simulink library "CarMaker4SL"  (Simulink 8.8)
settings: Solver=ode45  StartTime=0.0  StopTime=10.0  RelTol=1e-3
libraries: simulink x1
(part 1 of 2)
settings Model: Creator=fh  LastModifiedBy=Jeder  ExtModeAutoUpdateStatusClock=off

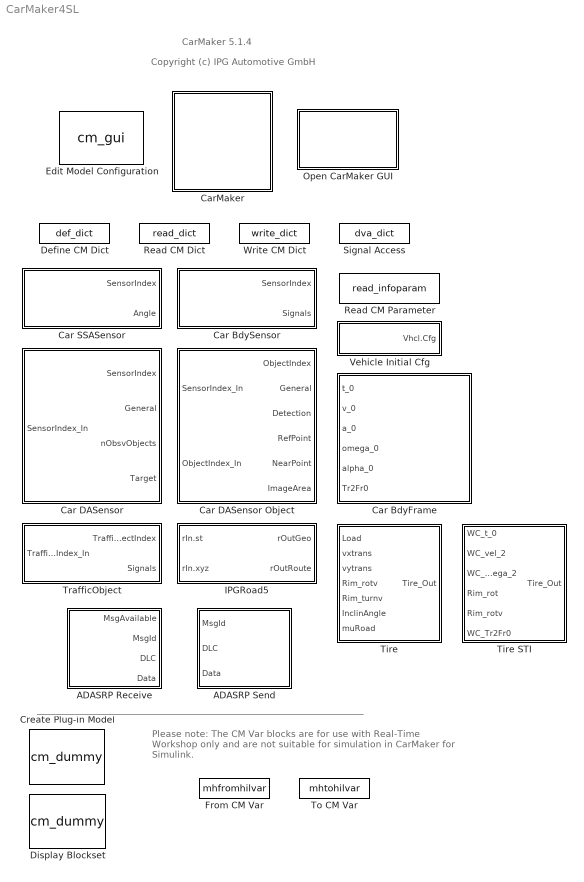
== system CarMaker4SL ==
  note: CarMaker 5.1.4
  note: Copyright (c) IPG Automotive GmbH
  note: ______________________________________________________________________
  note: Please note:
      | The CM Var blocks are for use with Real-Time Workshop only
      | and are not suitable for simulation in CarMaker for Simulink.
  ADASRP Receive : Subsystem  mask(ADASRP Receive){}
      mask help: Receive ADASP CAN message.
  ADASRP Send : Subsystem  mask(ADASRP Send){}
      mask help: Send ADASP CAN message.
  Car BdyFrame : Subsystem  mask(Body Frame){xname=[]}
      mask prompts: xname "BdyFrame name"
      mask help: Create a body frame on which sensors can be mounted.
      mask Display:
      | fprintf('<< %s >>', xname)
      | port_label('input', 1, 't_0')
      | port_label('input', 2, 'v_0')
      | port_label('input', 3, 'a_0')
      | port_label('input', 4, 'omega_0')
      | port_label('input', 5, 'alpha_0')
      | port_label('input', 6, 'Tr2Fr0')
  Car BdySensor : Subsystem  mask(CarMaker Bdy Sensor){xname=[]}
      mask prompts: xname "BdySensor name (or index)"
      mask help:
      | Read BdySensor.
      | The 'SensorIndex' outport shows either the sensor's internal index, or -1 if no BdySensor with the specified name exists.
      mask Display:
      | fprintf('<< %s >>', xname)
      | port_label('output', 1, 'SensorIndex')
      | port_label('output', 2, 'Signals')
  Car DASensor : Subsystem  mask(CarMaker Driving Assistance Sensor){xname=INPORT}
      mask prompts: xname "DASensor (name, index, or INPORT)"
      mask help:
      | Read Driving Assistance Sensor.
      | The sensor to be read may be specified in one of the following ways: 1. By giving the sensor's name. 2. By giving the sensor's numerical index. 3. By using the special name INPORT, so that the sensor's index is read from the 'si' inport.
      | The 'SensorIndex' outport shows either the sensor's index or -1 if no DASensor with the given name or index exists.
      mask Display:
      | fprintf('<< %s >>', xname)
      | port_label('input', 1, 'si')
      | port_label('output', 1, 'SensorIndex')
      | port_label('output', 2, 'General')
      | port_label('output', 3, 'nObsvObjects')
      | port_label('output', 4, 'Target')
  Car DASensor Object : Subsystem  mask(CarMaker Driving Assistance Sensor Object){xname=INPORT, ximode=Observed Objects}
      mask prompts: xname "DASensor Name (name, index, or INPORT)"; ximode "Addressed Objects"
      mask help:
      | Access sensor specific information about a traffic object.
      | The associated DASensor may be specified in one of the following ways: 1. By giving the sensor's name. 2. By giving the sensor's numerical index. 3. By using the special name INPORT, so that the sensor's index is read from the 'si' inport.
      | The object index is always read from the 'oi' inport. The 'ObjectIndex' outport shows either the object's index (world object index, see below) or -1 if no DASensor with the given name or index or no object at the given index exists.
      | You may use the special object index 99999 to select the sensor's relevant target object.
      | The object index addresses either one of the 'World Objects', i.e. all existing traffic objects, or one of the 'Observed Objects', i.e. the subset of objects inside the sensor's observation radius.
      mask TypeOptions ximode: Observed Objects | World Objects
      mask Display:
      | fprintf('<< %s >>', xname)
      | port_label('input', 1, 'si')
      | port_label('input', 2, 'oi')
      | port_label('output', 1, 'ObjectIndex')
      | port_label('output', 2, 'General')
      | port_label('output', 3, 'Detection')
      | port_label('output', 4, 'RefPoint')
      | port_label('output', 5, 'NearPoint')
      | port_label('output', 6, 'ImageArea')
  Car SSASensor : Subsystem  mask(CarMaker SideSlipAngle Sensor){xname=[]}
      mask prompts: xname "SSASensor name (or index)"
      mask help:
      | Read SideSlipAngle Sensor.
      | The 'SensorIndex' outport shows either the sensor's internal index, or -1 if no SSASensor with the specified name exists.
      mask Display:
      | fprintf('<< %s >>', xname)
      | port_label('output', 1, 'SensorIndex')
      | port_label('output', 2, 'Angle')
  CarMaker : Subsystem  TreatAsAtomicUnit=on
      mask Display: image(imread('CarMaker4SLss.bmp'));
  Create Plug-in Model : S-Function  FunctionName=cm_dummy  SFunctionDeploymentMode=off  EnableBusSupport=off  mask(Create CarMaker Plug-in Model){}
      settings: OpenFcn=cmPluginModel;
      mask Display: disp('Create\nCarMaker\nPlug-in Model');
  Define CM Dict : S-Function  FunctionName=def_dict  Parameters=xname, xunit, xmono,xtype,xnstates,xfirststate,xinitial,xdvaplace  SFunctionDeploymentMode=off  EnableBusSupport=off  mask(Define CarMaker Dictionary Variable){xname=, xunit=, xmono=off, xtype=Double4, xdvaplace=None, xnstates=0, xfirststate=0, xinitial=0}
      mask prompts: xname "Variable Name"; xunit "Unit"; xmono "Strictly monotone"; xtype "Type"; xdvaplace "DVA write access"; xnstates "Number of states (0=no states)"; xfirststate "First state (if number of states != 0)"; xinitial "Initial value"
      mask help: Define a new variable in the CarMaker data dictionary.
      mask TypeOptions xtype: Double | Double4 | Float | LLong | ULLong | Long | ULong | Int | UInt | Short | UShort | Char | UChar
      mask TypeOptions xdvaplace: None | IO_In | DM | VC | PTC | IO_Out | Private
      mask Display: disp(xname)
  Display Blockset : S-Function  FunctionName=cm_dummy  SFunctionDeploymentMode=off  EnableBusSupport=off
      settings: OpenFcn=open_system('CarMaker4SL')
      mask Display: disp('Display\nCarMaker4SL\nBlockset')
  Edit Model Configuration : S-Function  FunctionName=cm_gui  SFunctionDeploymentMode=off  EnableBusSupport=off
      settings: OpenFcn=cmmodelconf('edit');
      mask Display: disp('CarMaker\nModel\nConfiguration');
  From CM Var : S-Function  FunctionName=mhfromhilvar  Parameters=xname  SFunctionDeploymentMode=off  EnableBusSupport=off  mask(From CarMaker Var){xname=[]}
      mask prompts: xname "Variable Name"
      mask help:
      | Copy the value of the specified CarMaker C variable to the block's output port.
      |
      | PLEASE NOTE: This block is for use with Real-Time Workshop only, not for simulation in Simulink.
      mask Display: disp(xname)
  IPGRoad5 : Subsystem  mask(Query IPGRoad){xname=, xevalmode=GeoEval, xconsiderbumps=off, xusepath=off, xwithcurve=off, xabort=on}
      mask prompts: xname "Name"; xevalmode "Mode"; xconsiderbumps "Consider bumps"; xusepath "Use path"; xwithcurve "Output curvature"; xabort "Abort when off road"
      mask help:
      | Query IPGRoad about a given location.
      | The block should be given a unique name. In case of an error this name is logged together with the error message, making it easier to identify the location of the problem.
      mask TypeOptions xevalmode: GeoEval | RouteEval ST | RouteEval XY_S | RouteEval XY_SZ
      mask Display:
      | fprintf('<< %s >>\n%s', xname, xevalmode)
      | port_label('input', 1, 'st')
      | port_label('input', 2, 'xyz')
      | port_label('output', 1, 'Geo')
      | port_label('output', 2, 'Route')
  Open CarMaker GUI : Subsystem  LoadFcn=if ~length(which('cmcmd')), cmenv; end
      settings: OpenFcn=cmblockmagic('gui_fix_display'); CM_Simulink
      mask Display: image(imread('CarMakerGUI.bmp'));
  Read CM Dict : S-Function  FunctionName=read_dict  Parameters=xname, xsync  SFunctionDeploymentMode=off  EnableBusSupport=off  mask(Read CarMaker Dictionary Variable(s)){xname=, xsync=off}
      mask prompts: xname "Variable Name"; xsync "Show Sync Port"
      mask help: Copy the value(s) of the specified variable(s) of the CarMaker data dictionary to the block's output port(s). Separate the names of the variables with commas.
      mask Display: disp(xname)
  Read CM Parameter : S-Function  FunctionName=read_infoparam  Parameters=xfile,xkey,xnout,xdefaults,[],xmuxed  SFunctionDeploymentMode=off  EnableBusSupport=off  mask(Read CarMaker Infofile Parameter){xfile=Vehicle, xkey=Body.mass, xnout=1, xdefaults=0, xmuxed=on}
      mask prompts: xfile "Parameter location"; xkey "Parameter name"; xnout "Number of outputs"; xdefaults "Default value (scalar, vector [...], or empty matrix [ ])"; xmuxed "Muxed output"
      mask help: Read the first n elements of a CarMaker infofile parameter used in the current testrun. A default value may be provided in case the parameter does not exist or does not contain at least the specified number of elements. An empty matrix [ ] specified as the default value means the parameter must exist and contain the necessary number of element, otherwise an error is generated.
      mask TypeOptions xfile: SimParameters | ECUParameters | Testrun | Vehicle | VehicleExtraData | Aero | Brake | BrakeSystem | BrakeControl | Steering | SuspF | SuspR | SuspR2 | SuspF2 | SuspExtFrcs | TireFL | TireFR | TireRL | TireRR | TireRL2 | TireRR2 | TireFL2 | TireFR2 | PTControl | PTControlOSM | PowerTrain | PowerTrainXWD | PTEngineCU | PTEngine | PTMotorCU | PTMotorISG | PTMotor | PTMotor1 | PTMotor2 | PTMotor3 | PTMotor4 | PTMotor5 | PTMotor6 | PTMotor7 | PTTransmCU | PTClutch | PTGearBox | PTGearBoxM | PTGearBoxM1 | PTGearBoxM2 | PTGearBoxM3 | PTGearBoxM4 | PTGearBoxM5 | PTGearBoxM6 | PTGearBoxM7 | PTDriveLine | PTDriveLineXWD | PTBatteryCU | PTPowerSupply | PTGenCoupling_Front | PTGenCoupling_Rear | PTGenCoupling_Center | PTGenCoupling_Rear2 | PTGenCoupling_Front2 | PTGenCoupling_HangOn | PTGenCoupling_CenterFront | PTGenCoupling_CenterRear | UserDriver | VehicleControl | VhclOperator | Trailer | TrAero | TrBrake | TrBrakeSystem | TrBrakeControl | TrSuspF | TrSuspR | TrSuspM | TrSuspExtFrcs | TrTireFL | TrTireFR | TrTireRL | TrTireRR | TrTireML | TrTireMR | Trailer2 | Tr2Aero | Tr2Brake | Tr2BrakeSystem | Tr2BrakeControl | Tr2SuspF | Tr2SuspR | Tr2SuspM | Tr2SuspExtFrcs | Tr2TireFL | Tr2TireFR | Tr2TireRL | Tr2TireRR | Tr2TireML | Tr2TireMR
      mask Display: disp(sprintf('%s\n(%s)', xkey, xfile));
  Signal Access : S-Function  FunctionName=dva_dict  Parameters=xname, xunit, xmono,xtype,xnstates,xfirststate  SFunctionDeploymentMode=off  EnableBusSupport=off  mask(Add CarMaker DVA access to signal.){xname=, xunit=, xmono=off, xtype=Double4, xnstates=0, xfirststate=0}
      mask prompts: xname "Variable Name"; xunit "Unit"; xmono "Strictly monotone"; xtype "Type"; xnstates "Number of states (0=no states)"; xfirststate "First state (if number of states != 0)"
      mask help: The block's input is copied to its output, except when a DVA write access on the given dictionary variable is taking place, in which case the DVA value is copied. The quantity will always contain the signal's current value, so the block also provides a facility for quick signal inspection.
      mask TypeOptions xtype: Double | Double4 | Float | LLong | ULLong | Long | ULong | Int | UInt | Short | UShort | Char | UChar
      mask Display: disp(xname)
  Tire : Subsystem  mask(Tire){xtirepos=FL}
      mask prompts: xtirepos "Tire position"
      mask help:
      | Calculate Contact Point Interface (CPI) tire.
      | This block can only be used in a user defined vehicle.
      mask TypeOptions xtirepos: FL | FR | RL | RR
      mask Display:
      | port_label('input', 1, 'Load')
      | port_label('input', 2, 'vxtrans')
      | port_label('input', 3, 'vytrans')
      | port_label('input', 4, 'Rim_rotv')
      | port_label('input', 5, 'Rim_turnv')
      | port_label('input', 6, 'InclinAngle')
      | port_label('input', 7, 'muRoad')
      | port_label('output', 1, xtirepos)
  Tire STI : Subsystem  mask(Tire){xtirepos=FL}
      mask prompts: xtirepos "Tire position"
      mask help:
      | Calculate Standard Tire Interface (STI) tire.
      | This block can only be used in a user defined vehicle.
      mask TypeOptions xtirepos: FL | FR | RL | RR
      mask Display:
      | port_label('input', 1, 'WC_t_0')
      | port_label('input', 2, 'WC_vel_2')
      | port_label('input', 3, 'WC_omega_2')
      | port_label('input', 4, 'Rim_rot')
      | port_label('input', 5, 'Rim_rotv')
      | port_label('input', 6, 'WC_Tr2Fr0')
      | port_label('output', 1, xtirepos)
  To CM Var : S-Function  FunctionName=mhtohilvar  Parameters=xname  SFunctionDeploymentMode=off  EnableBusSupport=off  mask(To CarMaker Var){xname=[]}
      mask prompts: xname "Variable Name"
      mask help:
      | Copy the value of the block's input port to the specified CarMaker C variable.
      |
      | PLEASE NOTE: This block is for use with Real-Time Workshop only, not for simulation in Simulink.
      mask Display: disp(xname)
  TrafficObject : Subsystem  mask(CarMaker Traffic Object){xname=INPORT}
      mask prompts: xname "Traffic Object (name, index, or INPORT)"
      mask help:
      | Read Traffic Object.
      | The traffic object to be read may be specified in one of the following ways: 1. By giving the object's name. 2. By giving the object's numerical index. 3. By using the special name INPORT, so that the object's index is read from the 'toi' inport.
      | The 'TrafficObjectIndex' outport shows either the object's index or -1 if no traffic object with the given name or index exists.
      mask Display:
      | fprintf('<< %s >>', xname)
      | port_label('input', 1, 'toi')
      | port_label('output', 1, 'TrafficObjectIndex')
      | port_label('output', 2, 'TrafficObj')
  Vehicle Initial Cfg : Subsystem  mask(Vehicle Initial Configuration Values){}
      mask help: Provides some initial vehicle configuration values.
  Write CM Dict : S-Function  FunctionName=write_dict  Parameters=xname, xsync, 'off'  SFunctionDeploymentMode=off  EnableBusSupport=off  mask(Write CarMaker Dictionary Variable(s)){xname=, xsync=off}
      mask prompts: xname "Variable Name"; xsync "Show Sync Port"
      mask help: Copy the value(s) of the block's input port to the specified variable(s) of the CarMaker data dictionary. Separate the names of the variables with commas.
      mask Display: disp(xname)

== system CarMaker4SL/ADASRP Receive ==
  ADASRP Recv : S-Function  FunctionName=adasrp_recv  SFunctionDeploymentMode=off  EnableBusSupport=off
  MsgAvailable : Outport
  MsgId : Outport  Port=2
  DLC : Outport  Port=3
  Data : Outport  Port=4
  wires:
  ADASRP Recv/1 -> MsgAvailable/1
  ADASRP Recv/4 -> Data/1
  ADASRP Recv/2 -> MsgId/1
  ADASRP Recv/3 -> DLC/1

== system CarMaker4SL/ADASRP Send ==
  MsgId : Inport
  DLC : Inport  Port=2
  Data : Inport  Port=3
  ADASRP Send : S-Function  FunctionName=adasrp_send  SFunctionDeploymentMode=off  EnableBusSupport=off
  wires:
  MsgId/1 -> ADASRP Send/1
  DLC/1 -> ADASRP Send/2
  Data/1 -> ADASRP Send/3

== system CarMaker4SL/Car BdyFrame ==
  t_0 : Inport
  v_0 : Inport  Port=2
  a_0 : Inport  Port=3
  omega_0 : Inport  Port=4
  alpha_0 : Inport  Port=5
  Tr2Fr0 : Inport  Port=6
  S-Function : S-Function  FunctionName=cm_bdyframe  Parameters=xname  SFunctionDeploymentMode=off  EnableBusSupport=off
  wires:
  t_0/1 -> S-Function/1
  v_0/1 -> S-Function/2
  a_0/1 -> S-Function/3
  omega_0/1 -> S-Function/4
  alpha_0/1 -> S-Function/5
  Tr2Fr0/1 -> S-Function/6

== system CarMaker4SL/Car BdySensor ==
  Bus Creator1 : BusCreator  Inputs=38
  Demux1 : Demux  Outputs=38
  S-Function : S-Function  FunctionName=cm_bdysensor  Parameters=xname, 'unused'  SFunctionDeploymentMode=off  EnableBusSupport=off
  SensorIndex : Outport
  Signals : Outport  Port=2
  wires:
  S-Function/1 -> SensorIndex/1
  Demux1/1 -> Bus Creator1/1  "SignalMask"
  Demux1/2 -> Bus Creator1/2  "MountFrame"
  Demux1/3 -> Bus Creator1/3  "Pos_B x"
  Demux1/4 -> Bus Creator1/4  "Pos_B y"
  Demux1/5 -> Bus Creator1/5  "Pos_B z"
  Demux1/6 -> Bus Creator1/6  "Pos_0 x"
  Demux1/7 -> Bus Creator1/7  "Pos_0 y"
  Demux1/8 -> Bus Creator1/8  "Pos_0 z"
  Demux1/9 -> Bus Creator1/9  "Vel_B x"
  Demux1/10 -> Bus Creator1/10  "Vel_B y"
  Demux1/11 -> Bus Creator1/11  "Vel_B z"
  Demux1/12 -> Bus Creator1/12  "Vel_0 x"
  Demux1/13 -> Bus Creator1/13  "Vel_0 y"
  Demux1/14 -> Bus Creator1/14  "Vel_0 z"
  Demux1/15 -> Bus Creator1/15  "Acc_B x"
  Demux1/16 -> Bus Creator1/16  "Acc_B y"
  Demux1/17 -> Bus Creator1/17  "Acc_B z"
  Demux1/18 -> Bus Creator1/18  "Acc_0 x"
  Demux1/19 -> Bus Creator1/19  "Acc_0 y"
  Demux1/20 -> Bus Creator1/20  "Acc_0 z"
  Demux1/21 -> Bus Creator1/21  "Omega_B x"
  Demux1/22 -> Bus Creator1/22  "Omega_B y"
  Demux1/23 -> Bus Creator1/23  "Omega_B z"
  Demux1/24 -> Bus Creator1/24  "Omega_0 x"
  Demux1/25 -> Bus Creator1/25  "Omega_0 y"
  Demux1/26 -> Bus Creator1/26  "Omega_0 z"
  Demux1/27 -> Bus Creator1/27  "Alpha_B x"
  Demux1/28 -> Bus Creator1/28  "Alpha_B y"
  Demux1/29 -> Bus Creator1/29  "Alpha_B z"
  Demux1/30 -> Bus Creator1/30  "Alpha_0 x"
  Demux1/31 -> Bus Creator1/31  "Alpha_0 y"
  Demux1/32 -> Bus Creator1/32  "Alpha_0 z"
  Demux1/33 -> Bus Creator1/33  "OBO_B x"
  Demux1/34 -> Bus Creator1/34  "OBO_B y"
  Demux1/35 -> Bus Creator1/35  "OBO_B z"
  Demux1/36 -> Bus Creator1/36  "OBO_0 x"
  Demux1/37 -> Bus Creator1/37  "OBO_0 y"
  Demux1/38 -> Bus Creator1/38  "OBO_0 z"
  Bus Creator1/1 -> Signals/1
  S-Function/2 -> Demux1/1

== system CarMaker4SL/Car DASensor ==
  SensorIndex_In : Inport
  Bus Creator : BusCreator  Inputs=2
  Bus Creator2 : BusCreator  Inputs=8
  Demux : Demux  Outputs=2
  Demux2 : Demux  Outputs=8
  S-Function : S-Function  FunctionName=cm_dasensor  Parameters=xname  SFunctionDeploymentMode=off  EnableBusSupport=off
  SensorIndex : Outport
  General : Outport  Port=2
  nObsvObjects : Outport  Port=3
  Target : Outport  Port=4
  wires:
  Demux/2 -> Bus Creator/2  "relvTargetIndex"
  Demux/1 -> Bus Creator/1  "TargetDetected"
  S-Function/1 -> SensorIndex/1
  S-Function/4 -> Demux/1
  Bus Creator/1 -> Target/1
  S-Function/3 -> nObsvObjects/1
  Demux2/1 -> Bus Creator2/1  "TrackingType"
  S-Function/2 -> Demux2/1
  Bus Creator2/1 -> General/1
  Demux2/2 -> Bus Creator2/2  "Range"
  Demux2/3 -> Bus Creator2/3  "Alpha"
  Demux2/4 -> Bus Creator2/4  "Theta"
  Demux2/5 -> Bus Creator2/5  "Rot_zyx x"
  Demux2/6 -> Bus Creator2/6  "Rot_zyx y"
  Demux2/7 -> Bus Creator2/7  "Rot_zyx z"
  Demux2/8 -> Bus Creator2/8  "DrvLaneCurv"
  SensorIndex_In/1 -> S-Function/1

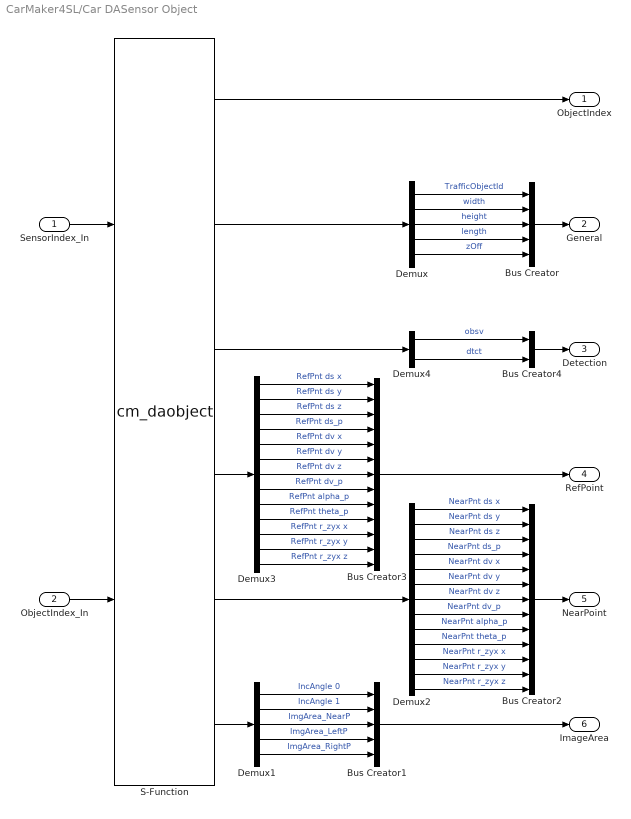
== system CarMaker4SL/Car DASensor Object ==
  SensorIndex_In : Inport
  ObjectIndex_In : Inport  Port=2
  Bus Creator : BusCreator  Inputs=5
  Bus Creator1 : BusCreator  Inputs=5
  Bus Creator2 : BusCreator  Inputs=13
  Bus Creator3 : BusCreator  Inputs=13
  Bus Creator4 : BusCreator  Inputs=2
  Demux : Demux  Outputs=5
  Demux1 : Demux  Outputs=5
  Demux2 : Demux  Outputs=13
  Demux3 : Demux  Outputs=13
  Demux4 : Demux  Outputs=2
  S-Function : S-Function  FunctionName=cm_daobject  Parameters=xname, ximode  SFunctionDeploymentMode=off  EnableBusSupport=off
  ObjectIndex : Outport
  General : Outport  Port=2
  Detection : Outport  Port=3
  RefPoint : Outport  Port=4
  NearPoint : Outport  Port=5
  ImageArea : Outport  Port=6
  wires:
  SensorIndex_In/1 -> S-Function/1
  ObjectIndex_In/1 -> S-Function/2
  Bus Creator4/1 -> Detection/1
  S-Function/3 -> Demux4/1
  S-Function/4 -> Demux3/1
  S-Function/5 -> Demux2/1
  S-Function/6 -> Demux1/1
  Demux4/2 -> Bus Creator4/2  "dtct"
  Demux4/1 -> Bus Creator4/1  "obsv"
  Bus Creator/1 -> General/1
  Demux/5 -> Bus Creator/5  "zOff"
  Demux/4 -> Bus Creator/4  "length"
  S-Function/2 -> Demux/1
  Demux2/10 -> Bus Creator2/10  "NearPnt theta_p"
  Bus Creator3/1 -> RefPoint/1
  Demux3/10 -> Bus Creator3/10  "RefPnt theta_p"
  Demux3/9 -> Bus Creator3/9  "RefPnt alpha_p"
  Demux3/8 -> Bus Creator3/8  "RefPnt dv_p"
  Demux3/7 -> Bus Creator3/7  "RefPnt dv z"
  Demux3/6 -> Bus Creator3/6  "RefPnt dv y"
  Demux3/5 -> Bus Creator3/5  "RefPnt dv x"
  Demux3/4 -> Bus Creator3/4  "RefPnt ds_p"
  Demux3/3 -> Bus Creator3/3  "RefPnt ds z"
  Demux3/2 -> Bus Creator3/2  "RefPnt ds y"
  Demux3/1 -> Bus Creator3/1  "RefPnt ds x"
  Bus Creator2/1 -> NearPoint/1
  Demux2/9 -> Bus Creator2/9  "NearPnt alpha_p"
  Demux2/8 -> Bus Creator2/8  "NearPnt dv_p"
  Demux2/7 -> Bus Creator2/7  "NearPnt dv z"
  Demux2/6 -> Bus Creator2/6  "NearPnt dv y"
  Demux2/5 -> Bus Creator2/5  "NearPnt dv x"
  Demux2/4 -> Bus Creator2/4  "NearPnt ds_p"
  Demux2/3 -> Bus Creator2/3  "NearPnt ds z"
  Demux2/2 -> Bus Creator2/2  "NearPnt ds y"
  Demux2/1 -> Bus Creator2/1  "NearPnt ds x"
  Bus Creator1/1 -> ImageArea/1
  Demux1/5 -> Bus Creator1/5  "ImgArea_RightP"
  Demux1/4 -> Bus Creator1/4  "ImgArea_LeftP"
  Demux1/3 -> Bus Creator1/3  "ImgArea_NearP"
  Demux1/2 -> Bus Creator1/2  "IncAngle 1"
  Demux1/1 -> Bus Creator1/1  "IncAngle 0"
  Demux/3 -> Bus Creator/3  "height"
  Demux/1 -> Bus Creator/1  "TrafficObjectId"
  S-Function/1 -> ObjectIndex/1
  Demux/2 -> Bus Creator/2  "width"
  Demux2/11 -> Bus Creator2/11  "NearPnt r_zyx x"
  Demux2/12 -> Bus Creator2/12  "NearPnt r_zyx y"
  Demux2/13 -> Bus Creator2/13  "NearPnt r_zyx z"
  Demux3/11 -> Bus Creator3/11  "RefPnt r_zyx x"
  Demux3/12 -> Bus Creator3/12  "RefPnt r_zyx y"
  Demux3/13 -> Bus Creator3/13  "RefPnt r_zyx z"

== system CarMaker4SL/Car SSASensor ==
  S-Function : S-Function  FunctionName=cm_ssasensor  Parameters=xname  SFunctionDeploymentMode=off  EnableBusSupport=off
  SensorIndex : Outport
  Angle : Outport  Port=2
  wires:
  S-Function/2 -> Angle/1
  S-Function/1 -> SensorIndex/1

== system CarMaker4SL/CarMaker ==
  CM_FIRST : Subsystem
  CM_LAST : Subsystem
  DrivMan : Subsystem
  Ground : Ground
  IPG Vehicle : Subsystem  TreatAsAtomicUnit=on
  Terminator : Terminator
  VehicleControl : Subsystem
  wires:
  VehicleControl/2(Vhcl.Model.Source) -> IPG Vehicle/2(Vhcl.Model.Source)
  VehicleControl/7(VhclCtrl.PT) -> IPG Vehicle/7(VhclCtrl.PT)
  VehicleControl/6(VhclCtrl.Brake) -> IPG Vehicle/6(VhclCtrl.Brake)
  VehicleControl/5(Vhcl.Misc) -> IPG Vehicle/5(Vhcl.Misc)
  VehicleControl/4(Vhcl.Wheel.In) -> IPG Vehicle/4(Vhcl.Wheel.In)
  VehicleControl/3(VhclCtrl.Steering) -> IPG Vehicle/3(VhclCtrl.Steering)
  VehicleControl/1(Sync_Out) -> IPG Vehicle/1(Sync_In)
  IPG Vehicle/1(Sync_Out) -> CM_LAST/1(Sync_In)
  Ground/1 -> CM_FIRST/1(Sync_In)
  CM_LAST/1(Sync_Out) -> Terminator/1
  CM_FIRST/1(Sync_Out) -> DrivMan/1(Sync_In)
  CM_FIRST/2(Env.Misc) -> DrivMan/2(Env.Misc)
  DrivMan/1(Sync_Out) -> VehicleControl/1(Sync_In)
  DrivMan/2(DrivMan.Out) -> VehicleControl/2(DrivMan.In)

== system CarMaker4SL/IPGRoad5 ==
  rIn.st : Inport
  rIn.xyz : Inport  Port=2
  Bus Creator1 : BusCreator  Inputs=9
  Bus Creator2 : BusCreator  Inputs=22
  Demux1 : Demux  Outputs=9
  Demux3 : Demux  Outputs=22
  S-Function : S-Function  FunctionName=cm_road  Parameters=xname,xevalmode,xconsiderbumps,xusepath,xwithcurve,xabort  SFunctionDeploymentMode=off  EnableBusSupport=off
  rOutGeo : Outport
  rOutRoute : Outport  Port=2
  wires:
  rIn.st/1 -> S-Function/1
  rIn.xyz/1 -> S-Function/2
  Bus Creator2/1 -> rOutRoute/1
  Demux3/1 -> Bus Creator2/1  "x"
  Demux3/2 -> Bus Creator2/2  "y"
  Demux3/3 -> Bus Creator2/3  "z"
  Demux3/4 -> Bus Creator2/4  "nuv x"
  Demux3/5 -> Bus Creator2/5  "nuv y"
  Demux3/6 -> Bus Creator2/6  "nuv z"
  Demux3/7 -> Bus Creator2/7  "suv x"
  Demux3/8 -> Bus Creator2/8  "suv y"
  Demux3/9 -> Bus Creator2/9  "suv z"
  Demux3/10 -> Bus Creator2/10  "tuv x"
  Demux3/11 -> Bus Creator2/11  "tuv y"
  Demux3/12 -> Bus Creator2/12  "tuv z"
  Demux3/14 -> Bus Creator2/14  "t"
  Demux3/13 -> Bus Creator2/13  "s"
  Demux3/15 -> Bus Creator2/15  "curveXY"
  Demux3/16 -> Bus Creator2/16  "width left"
  Demux3/17 -> Bus Creator2/17  "width right"
  Demux3/18 -> Bus Creator2/18  "onRoad"
  Demux3/19 -> Bus Creator2/19  "grade"
  Demux3/20 -> Bus Creator2/20  "slope"
  Demux3/21 -> Bus Creator2/21  "curveZ"
  Demux1/1 -> Bus Creator1/1  "x"
  Demux1/2 -> Bus Creator1/2  "y"
  Demux1/3 -> Bus Creator1/3  "z"
  Demux1/4 -> Bus Creator1/4  "nuv x"
  Demux1/5 -> Bus Creator1/5  "nuv y"
  Demux1/6 -> Bus Creator1/6  "nuv z"
  Demux1/7 -> Bus Creator1/7  "onRoad"
  Demux1/8 -> Bus Creator1/8  "onJunction"
  Demux1/9 -> Bus Creator1/9  "fric"
  Bus Creator1/1 -> rOutGeo/1
  S-Function/1 -> Demux1/1
  S-Function/2 -> Demux3/1
  Demux3/22 -> Bus Creator2/22  "fric"

== system CarMaker4SL/Open CarMaker GUI ==
  S-Function : S-Function  FunctionName=cm_gui  SFunctionDeploymentMode=off  EnableBusSupport=off

== system CarMaker4SL/Tire ==
  Load : Inport
  vxtrans : Inport  Port=2
  vytrans : Inport  Port=3
  Rim_rotv : Inport  Port=4
  Rim_turnv : Inport  Port=5
  InclinAngle : Inport  Port=6
  muRoad : Inport  Port=7
  Bus Creator : BusCreator  Inputs=11
  Demux1 : Demux  Outputs=11
  S-Function : S-Function  FunctionName=cm_tire  Parameters=xtirepos  SFunctionDeploymentMode=off  EnableBusSupport=off
  Tire_Out : Outport
  wires:
  Bus Creator/1 -> Tire_Out/1
  S-Function/1 -> Demux1/1
  Demux1/1 -> Bus Creator/1  "Slp"
  Demux1/2 -> Bus Creator/2  "Alpha"
  Demux1/3 -> Bus Creator/3  "TurnSlp"
  Demux1/4 -> Bus Creator/4  "rBelt_eff"
  Demux1/5 -> Bus Creator/5  "vBelt"
  Demux1/6 -> Bus Creator/6  "LongFrc"
  Demux1/7 -> Bus Creator/7  "SideFrc"
  Demux1/8 -> Bus Creator/8  "LoadFrc"
  Demux1/9 -> Bus Creator/9  "OverturnTrq"
  Demux1/10 -> Bus Creator/10  "RollResist"
  Demux1/11 -> Bus Creator/11  "AlignTrq"
  Load/1 -> S-Function/1
  vxtrans/1 -> S-Function/2
  vytrans/1 -> S-Function/3
  Rim_rotv/1 -> S-Function/4
  Rim_turnv/1 -> S-Function/5
  InclinAngle/1 -> S-Function/6
  muRoad/1 -> S-Function/7

== system CarMaker4SL/Tire STI ==
  WC_t_0 : Inport
  WC_vel_2 : Inport  Port=2
  WC_omega_2 : Inport  Port=3
  Rim_rot : Inport  Port=4
  Rim_rotv : Inport  Port=5
  WC_Tr2Fr0 : Inport  Port=6
  Bus Creator2 : BusCreator  Inputs=26
  Demux1 : Demux  Outputs=26
  S-Function : S-Function  FunctionName=cm_tire_sti  Parameters=xtirepos  SFunctionDeploymentMode=off  EnableBusSupport=off
  Tire_Out : Outport
  wires:
  Bus Creator2/1 -> Tire_Out/1
  S-Function/1 -> Demux1/1
  WC_Tr2Fr0/1 -> S-Function/6
  Rim_rotv/1 -> S-Function/5
  Rim_rot/1 -> S-Function/4
  WC_omega_2/1 -> S-Function/3
  WC_vel_2/1 -> S-Function/2
  WC_t_0/1 -> S-Function/1
  Demux1/26 -> Bus Creator2/26  "P_0 z"
  Demux1/25 -> Bus Creator2/25  "P_0 y"
  Demux1/24 -> Bus Creator2/24  "P_0 x"
  Demux1/23 -> Bus Creator2/23  "muRoad"
  Demux1/22 -> Bus Creator2/22  "Radius"
  Demux1/21 -> Bus Creator2/21  "rBelt_eff"
  Demux1/20 -> Bus Creator2/20  "vBelt"
  Demux1/19 -> Bus Creator2/19  "P_v0_W z"
  Demux1/18 -> Bus Creator2/18  "P_v0_W y"
  Demux1/17 -> Bus Creator2/17  "P_v0_W x"
  Demux1/16 -> Bus Creator2/16  "InclinAngle"
  Demux1/15 -> Bus Creator2/15  "TurnSlp"
  Demux1/14 -> Bus Creator2/14  "Alpha"
  Demux1/13 -> Bus Creator2/13  "Slp"
  Demux1/12 -> Bus Creator2/12  "Trq_W z"
  Demux1/11 -> Bus Creator2/11  "Trq_W y"
  Demux1/10 -> Bus Creator2/10  "Trq_W x"
  Demux1/9 -> Bus Creator2/9  "Frc_W z"
  Demux1/8 -> Bus Creator2/8  "Frc_W y"
  Demux1/7 -> Bus Creator2/7  "Frc_W x"
  Demux1/6 -> Bus Creator2/6  "Trq_C z"
  Demux1/5 -> Bus Creator2/5  "Trq_C y"
  Demux1/4 -> Bus Creator2/4  "Trq_C x"
  Demux1/3 -> Bus Creator2/3  "Frc_C z"
  Demux1/2 -> Bus Creator2/2  "Frc_C y"
  Demux1/1 -> Bus Creator2/1  "Frc_C x"

== system CarMaker4SL/TrafficObject ==
  TrafficObjectIndex_In : Inport
  Bus Creator : BusCreator  Inputs=29
  Demux : Demux  Outputs=29
  S-Function : S-Function  FunctionName=cm_obstacle  Parameters=xname  SFunctionDeploymentMode=off  EnableBusSupport=off
  TrafficObjectIndex : Outport
  Signals : Outport  Port=2
  wires:
  Demux/29 -> Bus Creator/29  "a_0 z"
  Demux/28 -> Bus Creator/28  "a_0 y"
  Demux/27 -> Bus Creator/27  "a_0 x"
  Demux/26 -> Bus Creator/26  "v_0 z"
  Demux/25 -> Bus Creator/25  "v_0 y"
  Demux/24 -> Bus Creator/24  "v_0 x"
  Demux/23 -> Bus Creator/23  "Tr2Fr0 2 2"
  Demux/22 -> Bus Creator/22  "Tr2Fr0 2 1"
  Demux/21 -> Bus Creator/21  "Tr2Fr0 2 0"
  Demux/20 -> Bus Creator/20  "Tr2Fr0 1 2"
  Demux/19 -> Bus Creator/19  "Tr2Fr0 1 1"
  Demux/18 -> Bus Creator/18  "Tr2Fr0 1 0"
  Demux/17 -> Bus Creator/17  "Tr2Fr0 0 2"
  Demux/16 -> Bus Creator/16  "Tr2Fr0 0 1"
  Demux/15 -> Bus Creator/15  "Tr2Fr0 0 0"
  Demux/14 -> Bus Creator/14  "r_zyx z"
  Demux/13 -> Bus Creator/13  "r_zyx y"
  Demux/12 -> Bus Creator/12  "r_zyx x"
  Demux/11 -> Bus Creator/11  "t_0 z"
  Demux/10 -> Bus Creator/10  "t_0 y"
  Demux/9 -> Bus Creator/9  "t_0 x"
  Demux/8 -> Bus Creator/8  "LatAcc"
  Demux/7 -> Bus Creator/7  "LatVel"
  Demux/6 -> Bus Creator/6  "LongAcc"
  Demux/5 -> Bus Creator/5  "LongVel"
  Demux/4 -> Bus Creator/4  "tRoad"
  Demux/3 -> Bus Creator/3  "sRoad"
  Demux/2 -> Bus Creator/2  "DetectLevel"
  Demux/1 -> Bus Creator/1  "State"
  Bus Creator/1 -> Signals/1
  S-Function/2 -> Demux/1
  TrafficObjectIndex_In/1 -> S-Function/1
  S-Function/1 -> TrafficObjectIndex/1

== system CarMaker4SL/Vehicle Initial Cfg ==
  CreateBus Vhcl.Cfg : Subsystem
  VehicleControlUpd : S-Function  FunctionName=cm_initial  SFunctionDeploymentMode=off  EnableBusSupport=off
  Vhcl.Cfg : Outport
  wires:
  CreateBus Vhcl.Cfg/1(Out1) -> Vhcl.Cfg/1
  VehicleControlUpd/1 -> CreateBus Vhcl.Cfg/1(In1)

== system CarMaker4SL/CarMaker/CM_FIRST ==
  Sync_In : Inport
  Bus Creator1 : BusCreator  Inputs=9
  Demux : Demux  Outputs=9
  Environment : S-Function  FunctionName=CM_Sfun  Parameters='Environment'  SFunctionDeploymentMode=off  EnableBusSupport=off
  IoIn : S-Function  FunctionName=CM_Sfun  Parameters='IoIn'  SFunctionDeploymentMode=off  EnableBusSupport=off
  Sync_Out : Outport
  Env.Misc : Outport  Port=2
  wires:
  Demux/9 -> Bus Creator1/9  "Env WindVel_tot z"
  Demux/8 -> Bus Creator1/8  "Env WindVel_tot y"
  Demux/7 -> Bus Creator1/7  "Env WindVel_tot x"
  Demux/6 -> Bus Creator1/6  "Env SolarRadiation"
  Demux/5 -> Bus Creator1/5  "Env Time"
  Sync_In/1 -> IoIn/1
  IoIn/1 -> Environment/1
  Environment/1 -> Sync_Out/1
  Demux/1 -> Bus Creator1/1  "Env Temperature"
  Demux/2 -> Bus Creator1/2  "Env AirDensity"
  Demux/3 -> Bus Creator1/3  "Env AirPressure"
  Demux/4 -> Bus Creator1/4  "Env AirHumidity"
  Environment/2 -> Demux/1
  Bus Creator1/1 -> Env.Misc/1

== system CarMaker4SL/CarMaker/CM_LAST ==
  Sync_In : Inport
  CM_User : S-Function  FunctionName=CM_Sfun  Parameters='CM_User'  SFunctionDeploymentMode=off  EnableBusSupport=off
  IoOut : S-Function  FunctionName=CM_Sfun  Parameters='IoOut'  SFunctionDeploymentMode=off  EnableBusSupport=off
  Sync_Out : Outport
  wires:
  Sync_In/1 -> CM_User/1
  CM_User/1 -> IoOut/1
  IoOut/1 -> Sync_Out/1

== system CarMaker4SL/CarMaker/DrivMan ==
  note: There's rarely a reason to override DrivMan signals.
      | Use the VehicleControl interface for this purpose.
  Sync_In : Inport
  Env.Misc : Inport  Port=2
  BusCreator : BusCreator  Inputs=17
  Demux : Demux  Outputs=17
  DrivMan : S-Function  FunctionName=CM_Sfun  Parameters='DrivMan'  SFunctionDeploymentMode=off  EnableBusSupport=off
  Sync_Out : Outport
  DrivMan.Out : Outport  Port=2
  wires:
  DrivMan/2 -> Demux/1
  BusCreator/1 -> DrivMan.Out/1
  DrivMan/1 -> Sync_Out/1
  Sync_In/1 -> DrivMan/1
  Env.Misc/1 -> DrivMan/2
  Demux/1 -> BusCreator/1  "DrivMan SST"
  Demux/2 -> BusCreator/2  "DrivMan Key"
  Demux/3 -> BusCreator/3  "DrivMan UserSignal0"
  Demux/4 -> BusCreator/4  "DrivMan UserSignal1"
  Demux/5 -> BusCreator/5  "DrivMan UserSignal2"
  Demux/6 -> BusCreator/6  "DrivMan UserSignal3"
  Demux/7 -> BusCreator/7  "DrivMan UserSignal4"
  Demux/8 -> BusCreator/8  "DrivMan SelectorCtrl"
  Demux/9 -> BusCreator/9  "DrivMan GearNo"
  Demux/10 -> BusCreator/10  "DrivMan Brake"
  Demux/11 -> BusCreator/11  "DrivMan BrakePark"
  Demux/12 -> BusCreator/12  "DrivMan Clutch"
  Demux/13 -> BusCreator/13  "DrivMan Gas"
  Demux/14 -> BusCreator/14  "DrivMan Steering Ang"
  Demux/15 -> BusCreator/15  "DrivMan Steering AngVel"
  Demux/16 -> BusCreator/16  "DrivMan Steering AngAcc"
  Demux/17 -> BusCreator/17  "DrivMan Steering Trq"

== system CarMaker4SL/CarMaker/IPG Vehicle ==
  Sync_In : Inport
  Vhcl.Model.Source : Inport  Port=2
  VhclCtrl.Steering : Inport  Port=3
  Vhcl.Wheel.In : Inport  Port=4
  Vhcl.Misc : Inport  Port=5
  VhclCtrl.Brake : Inport  Port=6
  VhclCtrl.PT : Inport  Port=7
  Brake : Subsystem
  CarAndTrailer : Subsystem
  PowerTrain : Subsystem
  Stop Simulation : Stop
  VehicleSource_BuiltIn : simulink/Logic and Bit Operations/Compare To Constant  relop=~=  const=1  OutDataTypeStr=boolean  ZeroCross=off
  Sync_Out : Outport
  wires:
  Brake/2(Vhcl.Wheel.PT) -> PowerTrain/2(Vhcl.Wheel.PT)
  VehicleSource_BuiltIn/1 -> Stop Simulation/1
  Vhcl.Model.Source/1 -> VehicleSource_BuiltIn/1
  Sync_In/1 -> CarAndTrailer/1(Sync_In)
  VhclCtrl.Steering/1 -> CarAndTrailer/2(VhclCtrl.Steering)
  Vhcl.Wheel.In/1 -> CarAndTrailer/3(Vhcl.Wheel.In)
  Vhcl.Misc/1 -> CarAndTrailer/4(Vhcl.Misc)
  PowerTrain/1(Sync_Out) -> Sync_Out/1
  VhclCtrl.Brake/1 -> Brake/3(VhclCtrl.Brake)
  CarAndTrailer/2(Brake.IF.In) -> Brake/2(Brake.IF.In)
  CarAndTrailer/1(Sync_Out) -> Brake/1(Sync_In)
  Brake/1(Sync_Out) -> PowerTrain/1(Sync_In)
  VhclCtrl.PT/1 -> PowerTrain/3(VhclCtrl.PT)

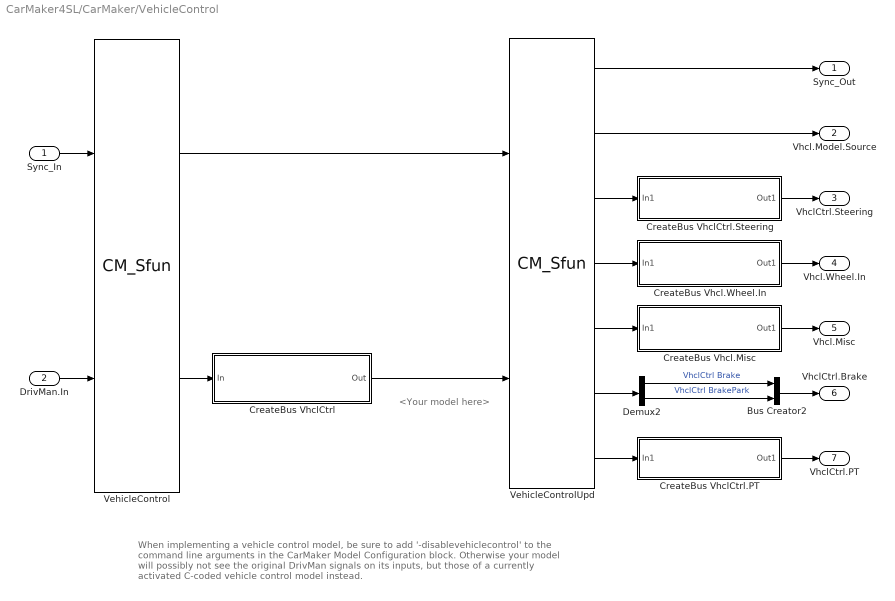
== system CarMaker4SL/CarMaker/VehicleControl ==
  note: When implementing a vehicle control model,
      | be sure to add '-disablevehiclecontrol' to the command line arguments
      | in the CarMaker Model Configuration block.
      | Otherwise your model will possibly not see the original DrivMan signals
      | on its inputs, but those of a currently activated C-coded vehicle control model instead.
  note: <Your model here>
  Sync_In : Inport
  DrivMan.In : Inport  Port=2
  Bus Creator2 : BusCreator  Inputs=2
  CreateBus Vhcl.Misc : Subsystem
  CreateBus Vhcl.Wheel.In : Subsystem
  CreateBus VhclCtrl : Subsystem
  CreateBus VhclCtrl.PT : Subsystem
  CreateBus VhclCtrl.Steering : Subsystem
  Demux2 : Demux  Outputs=2
  VehicleControl : S-Function  FunctionName=CM_Sfun  Parameters='VehicleControl'  SFunctionDeploymentMode=off  EnableBusSupport=off
  VehicleControlUpd : S-Function  FunctionName=CM_Sfun  Parameters='VehicleControlUpd'  SFunctionDeploymentMode=off  EnableBusSupport=off
  Sync_Out : Outport
  Vhcl.Model.Source : Outport  Port=2
  VhclCtrl.Steering : Outport  Port=3
  Vhcl.Wheel.In : Outport  Port=4
  Vhcl.Misc : Outport  Port=5
  VhclCtrl.Brake : Outport  Port=6
  VhclCtrl.PT : Outport  Port=7
  wires:
  Demux2/1 -> Bus Creator2/1  "VhclCtrl Brake"
  Demux2/2 -> Bus Creator2/2  "VhclCtrl BrakePark"
  VehicleControlUpd/1 -> Sync_Out/1
  CreateBus VhclCtrl.Steering/1(Out1) -> VhclCtrl.Steering/1
  Bus Creator2/1 -> VhclCtrl.Brake/1
  CreateBus VhclCtrl.PT/1(Out1) -> VhclCtrl.PT/1
  Sync_In/1 -> VehicleControl/1
  VehicleControl/1 -> VehicleControlUpd/1
  DrivMan.In/1 -> VehicleControl/2
  CreateBus Vhcl.Wheel.In/1(Out1) -> Vhcl.Wheel.In/1
  CreateBus Vhcl.Misc/1(Out1) -> Vhcl.Misc/1
  VehicleControlUpd/3 -> CreateBus VhclCtrl.Steering/1(In1)
  VehicleControlUpd/7 -> CreateBus VhclCtrl.PT/1(In1)
  VehicleControlUpd/6 -> Demux2/1
  VehicleControlUpd/5 -> CreateBus Vhcl.Misc/1(In1)
  VehicleControlUpd/4 -> CreateBus Vhcl.Wheel.In/1(In1)
  VehicleControlUpd/2 -> Vhcl.Model.Source/1
  VehicleControl/2 -> CreateBus VhclCtrl/1(In)
  CreateBus VhclCtrl/1(Out) -> VehicleControlUpd/2

== system CarMaker4SL/Vehicle Initial Cfg/CreateBus Vhcl.Cfg ==
  In1 : Inport
  Bus Creator : BusCreator  Inputs=13
  Demux : Demux  Outputs=13
  Out1 : Outport
  wires:
  Demux/3 -> Bus Creator/3  "Vhcl Cfg Fr1_Pos z"
  Demux/1 -> Bus Creator/1  "Vhcl Cfg Fr1_Pos x"
  Demux/2 -> Bus Creator/2  "Vhcl Cfg Fr1_Pos y"
  Demux/4 -> Bus Creator/4  "Vhcl Cfg Roll"
  Demux/5 -> Bus Creator/5  "Vhcl Cfg Yaw"
  Demux/6 -> Bus Creator/6  "Vhcl Cfg Pitch"
  Demux/7 -> Bus Creator/7  "Vhcl Cfg Engine_rotv"
  Demux/8 -> Bus Creator/8  "Vhcl Cfg GearBox_rotv_out"
  Demux/9 -> Bus Creator/9  "SimCore Trailer nTrailers"
  Demux/10 -> Bus Creator/10  "Vhcl Cfg Whl_rotv FL"
  Demux/11 -> Bus Creator/11  "Vhcl Cfg Whl_rotv FR"
  Demux/12 -> Bus Creator/12  "Vhcl Cfg Whl_rotv RL"
  In1/1 -> Demux/1
  Bus Creator/1 -> Out1/1
  Demux/13 -> Bus Creator/13  "Vhcl Cfg Whl_rotv RR"

== system CarMaker4SL/CarMaker/IPG Vehicle/Brake ==
  note: When replacing the entire braking system,
      | be sure to add '-disablebrake' to the command line arguments
      | in the CarMaker Model Configuration block.
  note: <Your model here>
  Sync_In : Inport
  Brake.IF.In : Inport  Port=2
  VhclCtrl.Brake : Inport  Port=3
  Brake : S-Function  FunctionName=CM_Sfun  Parameters='Brake'  SFunctionDeploymentMode=off  EnableBusSupport=off
  BrakeUpd : S-Function  FunctionName=CM_Sfun  Parameters='BrakeUpd'  SFunctionDeploymentMode=off  EnableBusSupport=off
  BusCreator : BusCreator  Inputs=12
  CreateBus Vhcl.Wheel.PT : Subsystem
  Demux : Demux  Outputs=12
  Sync_Out : Outport
  Vhcl.Wheel.PT : Outport  Port=2
  wires:
  CreateBus Vhcl.Wheel.PT/1(Out) -> Vhcl.Wheel.PT/1
  BrakeUpd/2 -> CreateBus Vhcl.Wheel.PT/1(In)
  Demux/1 -> BusCreator/1  "Brake IF Trq_WB FL"
  Demux/2 -> BusCreator/2  "Brake IF Trq_WB FR"
  Demux/3 -> BusCreator/3  "Brake IF Trq_WB RL"
  Demux/4 -> BusCreator/4  "Brake IF Trq_WB RR"
  Demux/5 -> BusCreator/5  "Brake IF Trq_PB FL"
  Demux/6 -> BusCreator/6  "Brake IF Trq_PB FR"
  Demux/7 -> BusCreator/7  "Brake IF Trq_PB RL"
  Demux/8 -> BusCreator/8  "Brake IF Trq_PB RR"
  Demux/9 -> BusCreator/9  "Brake IF Trq_Reg_trg FL"
  Demux/10 -> BusCreator/10  "Brake IF Trq_Reg_trg FR"
  Demux/11 -> BusCreator/11  "Brake IF Trq_Reg_trg RL"
  Demux/12 -> BusCreator/12  "Brake IF Trq_Reg_trg RR"
  Sync_In/1 -> Brake/1
  BusCreator/1 -> BrakeUpd/2
  Brake/2 -> Demux/1
  VhclCtrl.Brake/1 -> Brake/3
  Brake.IF.In/1 -> Brake/2
  Brake/1 -> BrakeUpd/1  "Sync"
  BrakeUpd/1 -> Sync_Out/1

== system CarMaker4SL/CarMaker/IPG Vehicle/CarAndTrailer ==
  Sync_In : Inport
  VhclCtrl.Steering : Inport  Port=2
  Vhcl.Wheel.In : Inport  Port=3
  Vhcl.Misc : Inport  Port=4
  CarAndTrailerUpd : Subsystem
  Forces : Subsystem
  Ground : Ground
  Kinematics : Subsystem
  Kinetics : Subsystem
  Steering : Subsystem
  Terminator : Terminator
  Terminator1 : Terminator
  Trailer : Subsystem
  Sync_Out : Outport
  Brake.IF.In : Outport  Port=2
  wires:
  Kinematics/9(lBuf) -> Forces/9(lBuf)
  Forces/12(FBuf) -> Kinetics/12(FBuf)
  Kinematics/8(lStabi) -> Forces/8(lStabi)
  Kinematics/1(Sync_Out) -> Forces/1(Sync_In)
  Kinematics/2(TireFL_In) -> Forces/2(TireFL_In)
  Kinematics/3(TireFR_In) -> Forces/3(TireFR_In)
  Kinematics/4(TireRL_In) -> Forces/4(TireRL_In)
  Kinematics/5(TireRR_In) -> Forces/5(TireRR_In)
  Forces/1(Sync_Out) -> Kinetics/1(Sync_In)
  Forces/3(Car.Aero) -> Kinetics/3(Car.Aero)
  Kinematics/7(vDamp) -> Forces/7(vDamp)
  Kinematics/6(lSpring) -> Forces/6(lSpring)
  Forces/2(Car.Virtual) -> Kinetics/2(Car.Virtual)
  Forces/4(Car.Load) -> Kinetics/4(Car.Load)
  Forces/5(TireFL_Out) -> Kinetics/5(TireFL.Out)
  Forces/6(TireFR_Out) -> Kinetics/6(TireFR.Out)
  Forces/7(TireRL_Out) -> Kinetics/7(TireRL.Out)
  Forces/8(TireRR_Out) -> Kinetics/8(TireRR.Out)
  Forces/9(FSpring) -> Kinetics/9(FSpring)
  Forces/10(FDamp) -> Kinetics/10(FDamp)
  Forces/11(FStabi) -> Kinetics/11(FStabi)
  Ground/1 -> CarAndTrailerUpd/10(Vhcl.Fr1A)
  Kinetics/1(Sync_Out) -> Trailer/1(Sync_In)
  Steering/1(Sync_Out) -> Kinematics/1(Sync_In)
  Sync_In/1 -> Steering/1(Sync_In)
  VhclCtrl.Steering/1 -> Steering/2(VhclCtrl.Steering)
  Kinetics/2(Trailer.Load) -> Trailer/2(Trailer.Load)
  Kinetics/3(Car.Hitch) -> Trailer/3(Car.Hitch)
  Kinetics/4(Car.Fr1) -> Trailer/4(Car.Fr1)
  Steering/2(Steer.IF) -> Kinematics/2(Steer.IF)
  Kinetics/5(Car.Trq_T2W) -> Trailer/5(Car.Trq_T2W)
  Kinetics/6(WheelCarrier.Misc) -> Trailer/6(WheelCarrier.Misc)
  Vhcl.Wheel.In/1 -> Terminator/1
  Vhcl.Misc/1 -> Terminator1/1
  CarAndTrailerUpd/1(Sync_Out) -> Sync_Out/1
  CarAndTrailerUpd/2(Brake.IF.In) -> Brake.IF.In/1
  Trailer/1(Sync_Out) -> CarAndTrailerUpd/1(Sync_In)
  Trailer/2(Vhcl.Steering) -> CarAndTrailerUpd/2(Vhcl.Steering)
  Trailer/3(Vhcl.Motion) -> CarAndTrailerUpd/3(Vhcl.Motion)
  Trailer/4(Vhcl.PoI) -> CarAndTrailerUpd/4(Vhcl.PoI)
  Trailer/5(Vhcl.Wheel.FL) -> CarAndTrailerUpd/5(Vhcl.Wheel.FL)
  Trailer/6(Vhcl.Wheel.FR) -> CarAndTrailerUpd/6(Vhcl.Wheel.FR)
  Trailer/7(Vhcl.Wheel.RL) -> CarAndTrailerUpd/7(Vhcl.Wheel.RL)
  Trailer/8(Vhcl.Wheel.RR) -> CarAndTrailerUpd/8(Vhcl.Wheel.RR)
  Trailer/9(Car.Hitch.FrcTrq) -> CarAndTrailerUpd/9(Car.Hitch.FrcTrq)

== system CarMaker4SL/CarMaker/IPG Vehicle/PowerTrain ==
  note: <Your model here>
  note: When replacing the entire powertrain,
      | be sure to add '-disablepowertrain' to the command line arguments
      | in the CarMaker Model Configuration block.
  Sync_In : Inport
  Vhcl.Wheel.PT : Inport  Port=2
  VhclCtrl.PT : Inport  Port=3
  BusCreator : BusCreator  Inputs=40
  Demux : Demux  Outputs=40
  PowerTrain : S-Function  FunctionName=CM_Sfun  Parameters='PowerTrain'  SFunctionDeploymentMode=off  EnableBusSupport=off
  PowerTrainUpd : S-Function  FunctionName=CM_Sfun  Parameters='PowerTrainUpd'  SFunctionDeploymentMode=off  EnableBusSupport=off
  Sync_Out : Outport
  wires:
  Vhcl.Wheel.PT/1 -> PowerTrain/2
  VhclCtrl.PT/1 -> PowerTrain/3
  Demux/40 -> BusCreator/40  "PT IF WRR Trq_BrakeReg_max"
  Demux/39 -> BusCreator/39  "PT IF WRR Trq_BrakeReg"
  Demux/38 -> BusCreator/38  "PT IF WRR Trq_Supp2WC"
  Demux/37 -> BusCreator/37  "PT IF WRR Trq_Drive"
  Demux/36 -> BusCreator/36  "PT IF WRR Trq_B2W"
  Demux/35 -> BusCreator/35  "PT IF WRR rotv"
  Demux/34 -> BusCreator/34  "PT IF WRR rot"
  Demux/33 -> BusCreator/33  "PT IF WRL Trq_BrakeReg_max"
  Demux/32 -> BusCreator/32  "PT IF WRL Trq_BrakeReg"
  Demux/31 -> BusCreator/31  "PT IF WRL Trq_Supp2WC"
  Demux/30 -> BusCreator/30  "PT IF WRL Trq_Drive"
  Demux/29 -> BusCreator/29  "PT IF WRL Trq_B2W"
  Demux/28 -> BusCreator/28  "PT IF WRL rotv"
  Demux/27 -> BusCreator/27  "PT IF WRL rot"
  Demux/26 -> BusCreator/26  "PT IF WFR Trq_BrakeReg_max"
  Demux/25 -> BusCreator/25  "PT IF WFR Trq_BrakeReg"
  Demux/24 -> BusCreator/24  "PT IF WFR Trq_Supp2WC"
  Demux/23 -> BusCreator/23  "PT IF WFR Trq_Drive"
  Demux/22 -> BusCreator/22  "PT IF WFR Trq_B2W"
  Demux/21 -> BusCreator/21  "PT IF WFR rotv"
  Demux/20 -> BusCreator/20  "PT IF WFR rot"
  Demux/19 -> BusCreator/19  "PT IF WFL Trq_BrakeReg_max"
  Demux/18 -> BusCreator/18  "PT IF WFL Trq_BrakeReg"
  Demux/17 -> BusCreator/17  "PT IF WFL Trq_Supp2WC"
  Demux/16 -> BusCreator/16  "PT IF WFL Trq_Drive"
  Demux/15 -> BusCreator/15  "PT IF WFL Trq_B2W"
  Demux/14 -> BusCreator/14  "PT IF WFL rotv"
  Demux/13 -> BusCreator/13  "PT IF WFL rot"
  Demux/12 -> BusCreator/12  "PT IF DL_iDiff_mean"
  Demux/11 -> BusCreator/11  "PT IF Trq_Supp2BdyEng y"
  Demux/10 -> BusCreator/10  "PT IF Trq_Supp2BdyEng x"
  Demux/9 -> BusCreator/9  "PT IF Trq_Supp2Bdy1 z"
  Demux/8 -> BusCreator/8  "PT IF Trq_Supp2Bdy1 y"
  Demux/7 -> BusCreator/7  "PT IF Trq_Supp2Bdy1 x"
  Demux/6 -> BusCreator/6  "PT IF Engine_Trq (EngineControl)"
  Demux/5 -> BusCreator/5  "PT IF Engine_rotv"
  Demux/4 -> BusCreator/4  "PT IF GearNo"
  Demux/3 -> BusCreator/3  "PT IF OperationError"
  Demux/2 -> BusCreator/2  "PT IF OperationState"
  Demux/1 -> BusCreator/1  "PT IF Ignition"
  BusCreator/1 -> PowerTrainUpd/2
  PowerTrain/1 -> PowerTrainUpd/1  "Sync"
  PowerTrainUpd/1 -> Sync_Out/1
  PowerTrain/2 -> Demux/1
  Sync_In/1 -> PowerTrain/1

== system CarMaker4SL/CarMaker/VehicleControl/CreateBus Vhcl.Misc ==
  In1 : Inport
  Bus Creator5 : BusCreator  Inputs=11
  Demux5 : Demux  Outputs=11
  Out1 : Outport
  wires:
  Demux5/1 -> Bus Creator5/1  "Vhcl Trq_DL2Bdy1 x"
  Demux5/2 -> Bus Creator5/2  "Vhcl Trq_DL2Bdy1 y"
  Bus Creator5/1 -> Out1/1
  In1/1 -> Demux5/1
  Demux5/3 -> Bus Creator5/3  "Vhcl Trq_DL2Bdy1 z"
  Demux5/4 -> Bus Creator5/4  "Vhcl TrqDL2Bdy1B x"
  Demux5/5 -> Bus Creator5/5  "Vhcl TrqDL2Bdy1B y"
  Demux5/6 -> Bus Creator5/6  "Vhcl TrqDL2Bdy1B z"
  Demux5/7 -> Bus Creator5/7  "Vhcl DL2BdyEng x"
  Demux5/8 -> Bus Creator5/8  "Vhcl DL2BdyEng y"
  Demux5/9 -> Bus Creator5/9  "Vhcl Wind_vel_0 x"
  Demux5/10 -> Bus Creator5/10  "Vhcl Wind_vel_0 y"
  Demux5/11 -> Bus Creator5/11  "Vhcl Wind_vel_0 z"

== system CarMaker4SL/CarMaker/VehicleControl/CreateBus Vhcl.Wheel.In ==
  In1 : Inport
  Bus Creator1 : BusCreator  Inputs=12
  Demux1 : Demux  Outputs=12
  Out1 : Outport
  wires:
  Demux1/1 -> Bus Creator1/1  "Vhcl Wheel FL Trq_B2WC"
  Demux1/2 -> Bus Creator1/2  "Vhcl Wheel FL Trq_DL2WC"
  Bus Creator1/1 -> Out1/1
  In1/1 -> Demux1/1
  Demux1/3 -> Bus Creator1/3  "Vhcl Wheel FL rotv"
  Demux1/4 -> Bus Creator1/4  "Vhcl Wheel FR Trq_B2WC"
  Demux1/5 -> Bus Creator1/5  "Vhcl Wheel FR Trq_DL2WC"
  Demux1/6 -> Bus Creator1/6  "Vhcl Wheel FR rotv"
  Demux1/7 -> Bus Creator1/7  "Vhcl Wheel RL Trq_B2WC"
  Demux1/8 -> Bus Creator1/8  "Vhcl Wheel RL Trq_DL2WC"
  Demux1/9 -> Bus Creator1/9  "Vhcl Wheel RL rotv"
  Demux1/10 -> Bus Creator1/10  "Vhcl Wheel RR Trq_B2WC"
  Demux1/11 -> Bus Creator1/11  "Vhcl Wheel RR Trq_DL2WC"
  Demux1/12 -> Bus Creator1/12  "Vhcl Wheel RR rotv"

== system CarMaker4SL/CarMaker/VehicleControl/CreateBus VhclCtrl ==
  In : Inport
  BusCreator : BusCreator  Inputs=29
  Demux : Demux  Outputs=29
  Out : Outport
  wires:
  Demux/29 -> BusCreator/29  "VhclCtrl Lights Reverse"
  Demux/28 -> BusCreator/28  "VhclCtrl Lights Brake"
  Demux/27 -> BusCreator/27  "VhclCtrl Lights FogRear"
  Demux/26 -> BusCreator/26  "VhclCtrl Lights FogFrontR"
  Demux/25 -> BusCreator/25  "VhclCtrl Lights FogFrontL"
  Demux/24 -> BusCreator/24  "VhclCtrl Lights IndR"
  Demux/23 -> BusCreator/23  "VhclCtrl Lights IndL"
  Demux/22 -> BusCreator/22  "VhclCtrl Lights ParkR"
  Demux/21 -> BusCreator/21  "VhclCtrl Lights ParkL"
  Demux/20 -> BusCreator/20  "VhclCtrl Lights Daytime"
  Demux/19 -> BusCreator/19  "VhclCtrl Lights HighBeam"
  Demux/18 -> BusCreator/18  "VhclCtrl Lights LowBeam"
  Demux/17 -> BusCreator/17  "VhclCtrl Steering Trq"
  Demux/16 -> BusCreator/16  "VhclCtrl Steering AngAcc"
  Demux/15 -> BusCreator/15  "VhclCtrl Steering AngVel"
  Demux/14 -> BusCreator/14  "VhclCtrl Steering Ang"
  Demux/13 -> BusCreator/13  "VhclCtrl Gas"
  Demux/12 -> BusCreator/12  "VhclCtrl Clutch"
  Demux/11 -> BusCreator/11  "VhclCtrl BrakePark"
  Demux/10 -> BusCreator/10  "VhclCtrl Brake"
  Demux/9 -> BusCreator/9  "VhclCtrl SelectorCtrl"
  Demux/8 -> BusCreator/8  "VhclCtrl GearNo"
  Demux/7 -> BusCreator/7  "VhclCtrl UserSignal4"
  Demux/6 -> BusCreator/6  "VhclCtrl UserSignal3"
  Demux/5 -> BusCreator/5  "VhclCtrl UserSignal2"
  Demux/4 -> BusCreator/4  "VhclCtrl UserSignal1"
  Demux/3 -> BusCreator/3  "VhclCtrl UserSignal0"
  Demux/2 -> BusCreator/2  "VhclCtrl Key"
  Demux/1 -> BusCreator/1  "VhclCtrl SST"
  BusCreator/1 -> Out/1
  In/1 -> Demux/1

== system CarMaker4SL/CarMaker/VehicleControl/CreateBus VhclCtrl.PT ==
  In1 : Inport
  BusCreator : BusCreator  Inputs=11
  Demux : Demux  Outputs=11
  Out1 : Outport
  wires:
  Demux/11 -> BusCreator/11  "VhclCtrl Gas"
  Demux/10 -> BusCreator/10  "VhclCtrl Clutch"
  Demux/9 -> BusCreator/9  "VhclCtrl SelectorCtrl"
  Demux/8 -> BusCreator/8  "VhclCtrl GearNo"
  Demux/7 -> BusCreator/7  "VhclCtrl UserSignal4"
  Demux/6 -> BusCreator/6  "VhclCtrl UserSignal3"
  Demux/5 -> BusCreator/5  "VhclCtrl UserSignal2"
  Demux/4 -> BusCreator/4  "VhclCtrl UserSignal1"
  Demux/3 -> BusCreator/3  "VhclCtrl UserSignal0"
  Demux/2 -> BusCreator/2  "VhclCtrl Key"
  Demux/1 -> BusCreator/1  "VhclCtrl SST"
  BusCreator/1 -> Out1/1
  In1/1 -> Demux/1

== system CarMaker4SL/CarMaker/VehicleControl/CreateBus VhclCtrl.Steering ==
  In1 : Inport
  Bus Creator : BusCreator  Inputs=5
  Demux : Demux  Outputs=5
  Out1 : Outport
  wires:
  Demux/4 -> Bus Creator/4  "VhclCtrl Steering Trq"
  Demux/2 -> Bus Creator/2  "VhclCtrl Steering AngVel"
  Demux/3 -> Bus Creator/3  "VhclCtrl Steering AngAcc"
  Demux/5 -> Bus Creator/5  "VhclCtrl Steering ByTrq"
  Demux/1 -> Bus Creator/1  "VhclCtrl Steering Ang"
  Bus Creator/1 -> Out1/1
  In1/1 -> Demux/1

== system CarMaker4SL/CarMaker/IPG Vehicle/Brake/CreateBus Vhcl.Wheel.PT ==
  In : Inport
  BusCreator : BusCreator  Inputs=16
  Demux : Demux  Outputs=16
  Out : Outport
  wires:
  In/1 -> Demux/1
  BusCreator/1 -> Out/1
  Demux/1 -> BusCreator/1  "Vhcl Wheel FL Trq_Brake"
  Demux/2 -> BusCreator/2  "Vhcl Wheel FL Trq_BrakeReg_trg"
  Demux/3 -> BusCreator/3  "Vhcl Wheel FL Trq_T2W"
  Demux/4 -> BusCreator/4  "Vhcl Wheel FL WhlBearing"
  Demux/5 -> BusCreator/5  "Vhcl Wheel FR Trq_Brake"
  Demux/6 -> BusCreator/6  "Vhcl Wheel FR Trq_BrakeReg_trg"
  Demux/7 -> BusCreator/7  "Vhcl Wheel FR Trq_T2W"
  Demux/8 -> BusCreator/8  "Vhcl Wheel FR WhlBearing"
  Demux/9 -> BusCreator/9  "Vhcl Wheel RL Trq_Brake"
  Demux/10 -> BusCreator/10  "Vhcl Wheel RL Trq_BrakeReg_trg"
  Demux/11 -> BusCreator/11  "Vhcl Wheel RL Trq_T2W"
  Demux/12 -> BusCreator/12  "Vhcl Wheel RL WhlBearing"
  Demux/13 -> BusCreator/13  "Vhcl Wheel RR Trq_Brake"
  Demux/14 -> BusCreator/14  "Vhcl Wheel RR Trq_BrakeReg_trg"
  Demux/15 -> BusCreator/15  "Vhcl Wheel RR Trq_T2W"
  Demux/16 -> BusCreator/16  "Vhcl Wheel RR WhlBearing"
